simulink library "ad_mem_base"  (R2017a)
settings: Solver=VariableStepAuto  StartTime=0.0  StopTime=10.0  RelTol=1e-3
settings Model: Creator=eruffaldi  LastModifiedBy=eruffaldi

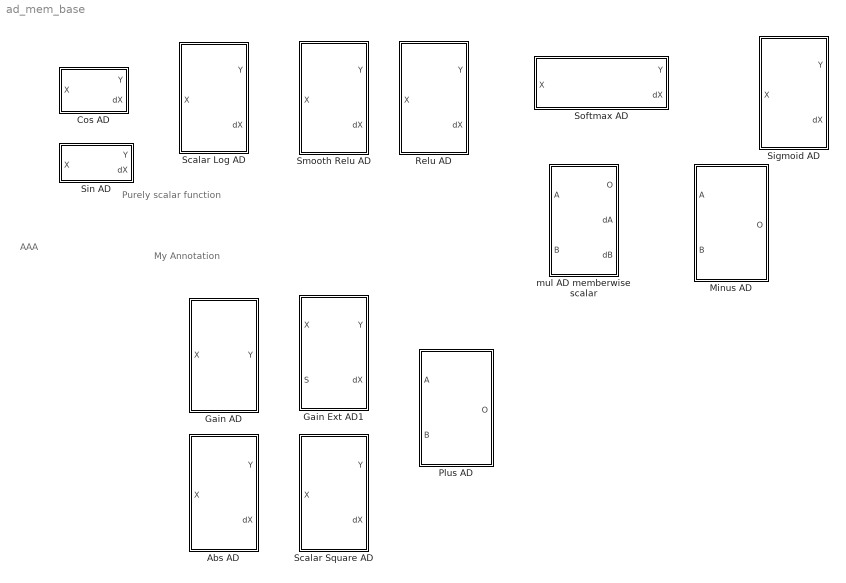
== system ad_mem_base ==
  note: AAA
  note: My Annotation
  note: Purely scalar function
  Abs AD : Subsystem
  Cos AD : Subsystem
  Gain AD : Subsystem  mask{k=1}
      mask prompts: k "Gain Constant"
  Gain Ext AD1 : Subsystem
  Minus AD : Subsystem
  "Plus AD " : Subsystem
  Relu AD : Subsystem
  Scalar Log AD : Subsystem
  Scalar Square AD : Subsystem
  Sigmoid AD : Subsystem
  Sin AD : Subsystem
  Smooth Relu AD : Subsystem
  Softmax AD : Subsystem
      mask Display: image('softmax.png');
  mul AD memberwise scalar : Subsystem

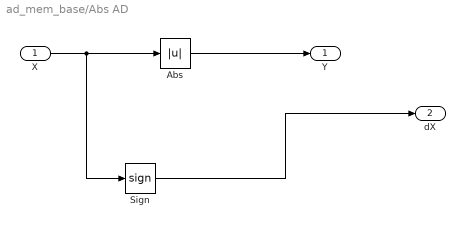
== system ad_mem_base/Abs AD ==
  X : Inport
  Abs : Abs
  Sign : Signum
  Y : Outport
  dX : Outport  Port=2
  wires:
  Abs/1 -> Y/1
  X/1 -> Sign/1, Abs/1
  Sign/1 -> dX/1

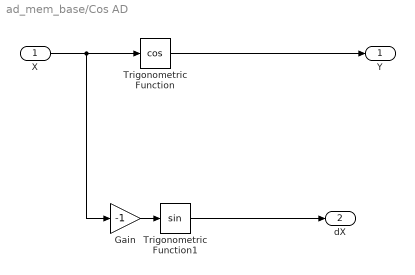
== system ad_mem_base/Cos AD ==
  X : Inport
  Gain : Gain  Gain=-1
  Trigonometric Function : Trigonometry  Operator=cos
  Trigonometric Function1 : Trigonometry
  Y : Outport
  dX : Outport  Port=2
  wires:
  Trigonometric Function/1 -> Y/1
  X/1 -> Gain/1, Trigonometric Function/1
  Gain/1 -> Trigonometric Function1/1
  Trigonometric Function1/1 -> dX/1

== system ad_mem_base/Gain AD ==
  X : Inport
  Gain1 : Gain  Gain=k
  Y : Outport
  wires:
  Gain1/1 -> Y/1
  X/1 -> Gain1/1

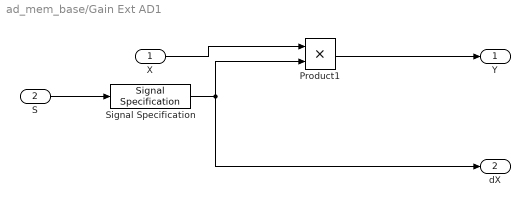
== system ad_mem_base/Gain Ext AD1 ==
  X : Inport
  S : Inport  Port=2
  Product1 : Product
  Signal Specification : SignalSpecification  Dimensions=1
  Y : Outport
  dX : Outport  Port=2
  wires:
  Product1/1 -> Y/1
  X/1 -> Product1/1
  Signal Specification/1 -> dX/1, Product1/2
  S/1 -> Signal Specification/1

== system ad_mem_base/Minus AD ==
  A : Inport
  B : Inport  Port=2
  Add : Sum  Inputs=+-
  O : Outport
  wires:
  Add/1 -> O/1
  A/1 -> Add/1
  B/1 -> Add/2

== system ad_mem_base/Plus AD  ==
  A : Inport
  B : Inport  Port=2
  Add : Sum
  O : Outport
  wires:
  Add/1 -> O/1
  A/1 -> Add/1
  B/1 -> Add/2

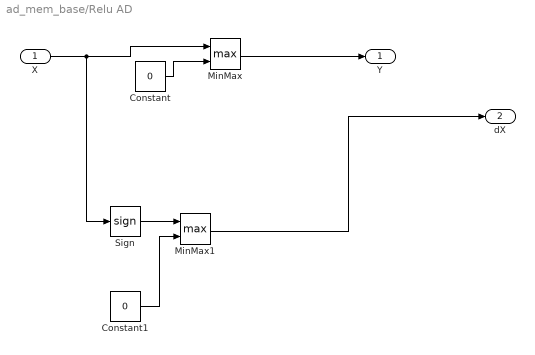
== system ad_mem_base/Relu AD ==
  X : Inport
  Constant : Constant  Value=0
  Constant1 : Constant  Value=0
  MinMax : MinMax  Function=max  Inputs=2
  MinMax1 : MinMax  Function=max  Inputs=2
  Sign : Signum
  Y : Outport
  dX : Outport  Port=2
  wires:
  MinMax/1 -> Y/1
  X/1 -> Sign/1, MinMax/1
  Constant/1 -> MinMax/2
  Sign/1 -> MinMax1/1
  Constant1/1 -> MinMax1/2
  MinMax1/1 -> dX/1

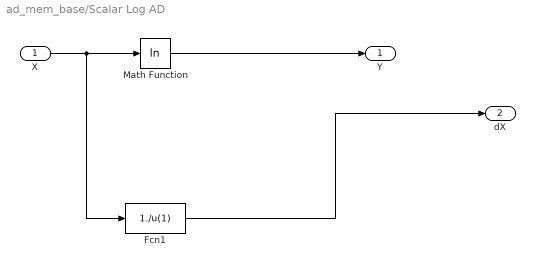
== system ad_mem_base/Scalar Log AD ==
  X : Inport
  Fcn1 : Fcn  Expr=1./u(1)
  Math Function : Math  Operator=log  SaturateOnIntegerOverflow=on
  Y : Outport
  dX : Outport  Port=2
  wires:
  Math Function/1 -> Y/1
  X/1 -> Fcn1/1, Math Function/1
  Fcn1/1 -> dX/1

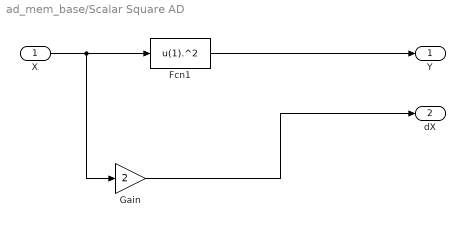
== system ad_mem_base/Scalar Square AD ==
  X : Inport
  Fcn1 : Fcn  Expr=u(1).^2
  Gain : Gain  Gain=2
  Y : Outport
  dX : Outport  Port=2
  wires:
  Fcn1/1 -> Y/1
  X/1 -> Gain/1, Fcn1/1
  Gain/1 -> dX/1

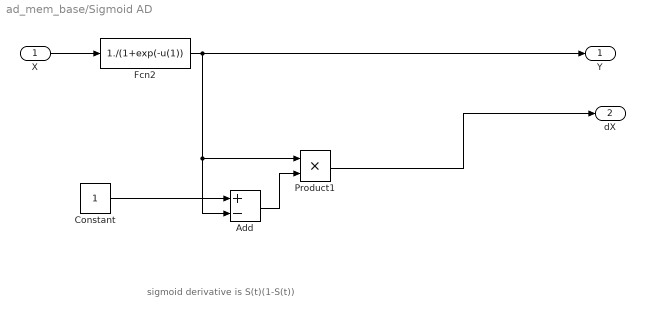
== system ad_mem_base/Sigmoid AD ==
  note: sigmoid derivative is S(t)(1-S(t))
  X : Inport
  Add : Sum  Inputs=+-
  Constant : Constant
  Fcn2 : Fcn  Expr=1./(1+exp(-u(1))
  Product1 : Product
  Y : Outport
  dX : Outport  Port=2
  wires:
  X/1 -> Fcn2/1
  Fcn2/1 -> Add/2, Product1/1, Y/1
  Constant/1 -> Add/1
  Add/1 -> Product1/2
  Product1/1 -> dX/1

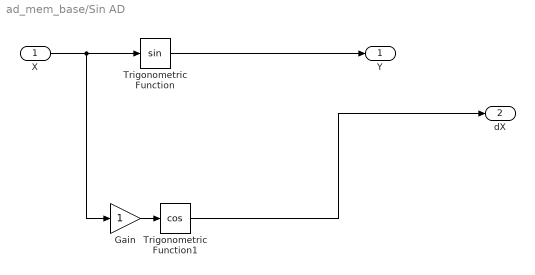
== system ad_mem_base/Sin AD ==
  X : Inport
  Gain : Gain
  Trigonometric Function : Trigonometry
  Trigonometric Function1 : Trigonometry  Operator=cos
  Y : Outport
  dX : Outport  Port=2
  wires:
  Trigonometric Function/1 -> Y/1
  X/1 -> Gain/1, Trigonometric Function/1
  Gain/1 -> Trigonometric Function1/1
  Trigonometric Function1/1 -> dX/1

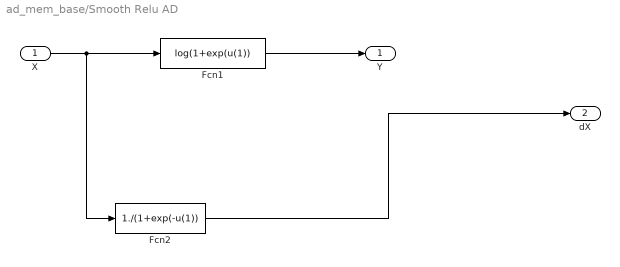
== system ad_mem_base/Smooth Relu AD ==
  X : Inport
  Fcn1 : Fcn  Expr=log(1+exp(u(1))
  Fcn2 : Fcn  Expr=1./(1+exp(-u(1))
  Y : Outport
  dX : Outport  Port=2
  wires:
  Fcn1/1 -> Y/1
  X/1 -> Fcn2/1, Fcn1/1
  Fcn2/1 -> dX/1

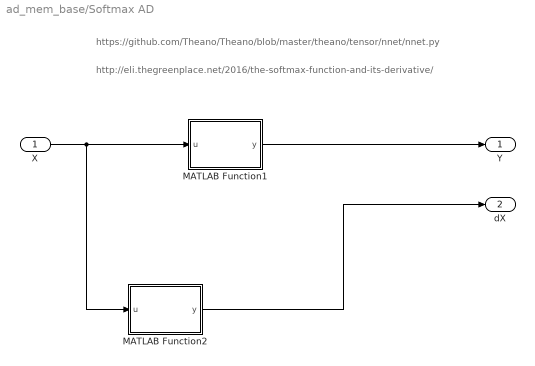
== system ad_mem_base/Softmax AD ==
  note: https://github.com/Theano/Theano/blob/master/theano/tensor/nnet/nnet.py
  note: http://eli.thegreenplace.net/2016/the-softmax-function-and-its-derivative/
  X : Inport
  MATLAB Function1 : MATLAB Function  TreatAsAtomicUnit=on
  MATLAB Function2 : MATLAB Function  TreatAsAtomicUnit=on
  Y : Outport
  dX : Outport  Port=2
  wires:
  MATLAB Function1/1(y) -> Y/1
  X/1 -> MATLAB Function2/1(u), MATLAB Function1/1(u)
  MATLAB Function2/1(y) -> dX/1

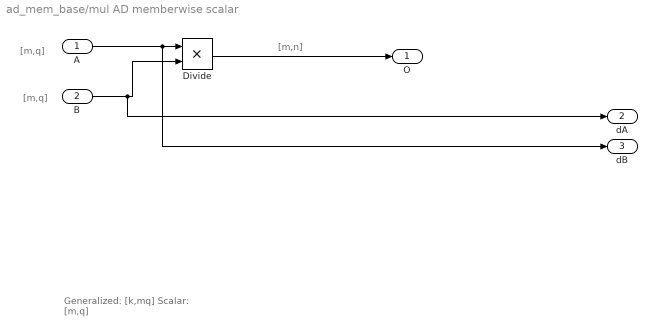
== system ad_mem_base/mul AD memberwise scalar ==
  note: Generalized: [k,mq]
      | Scalar: [m,q]
  note: [m,q]
  note: [m,q]
  note: [m,n]
  A : Inport
  B : Inport  Port=2
  Divide : Product  Inputs=**
  O : Outport
  dA : Outport  Port=2
  dB : Outport  Port=3
  wires:
  B/1 -> dA/1, Divide/2
  A/1 -> dB/1, Divide/1
  Divide/1 -> O/1

== matlab function ad_mem_base/Softmax AD/MATLAB Function1 ==
  data: u input; y output
function y = fcn(u)
%#codegen
exps = exp(u-max(u(:)));
y = exps/sum(exps(:));

== matlab function ad_mem_base/Softmax AD/MATLAB Function2 ==
  data: u input; y output
function y = fcn(u)

y = 1./(1+exp(-u));
